simulink model "LIB_CoffeeMachine"  (R2024b)
settings: Solver=FixedStepAuto  StartTime=0.0  StopTime=10.0  FixedStep=0.1  RelTol=1e-3
libraries: simulink_extras x1
settings Model: Creator=RAPQ2Y  LastModifiedBy=RAPQ2Y
settings HardwareCC: ProdBitPerPointer=32  ProdBitPerSizeT=32  ProdBitPerPtrDiffT=32  ProdWordSize=32  ProdLongLongMode=on  ProdHWDeviceType=PHOENIX CONTACT->Generic PLCnext 32bit  TargetPreprocMaxBitsSint=64  TargetPreprocMaxBitsUint=64
settings SFSimCC: MATLABDynamicMemAlloc=off
settings RTWCC: Description=PLCnext Target for Simulink for GRT purpose  SystemTargetFile=pxc_plcn.tlc  TLCOptions=-m1 -p10000000000000000000  TemplateMakefile=pxc_plcn__2020b.tmf  TargetLang=C++
settings CodeAppCC: MaxIdLength=63
settings STFCustomTargetCC: TargetLibSuffix=.a  TargetLangStandard=C++03 (ISO)  CodeReplacementLibrary=GNU C99 extensions  ParMdlRefBuildCompliant=on  ConcurrentExecutionCompliant=on  CombineOutputUpdateFcns=on  SystemTargetFile=pxc_plcn.tlc
settings GRTTargetCC: TargetLibSuffix=.a  TargetLangStandard=C++03 (ISO)  CodeReplacementLibrary=GNU C99 extensions  CompOptLevelCompliant=off  MatFileLogging=off  CPPClassGenCompliant=off  UseToolchainInfoCompliant=off  ExtModeMexFile=ext_comm_plcn

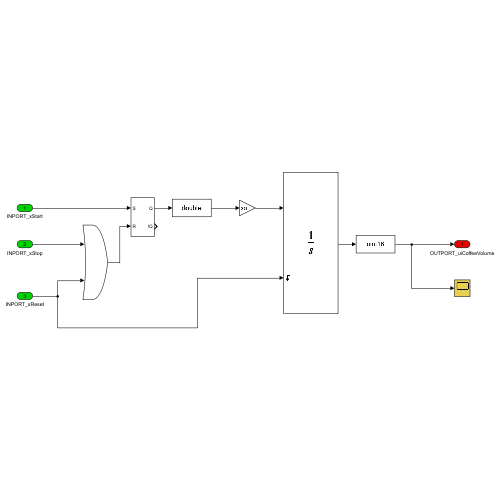
[thumbnail: Simulink's stored preview of the top-level diagram]
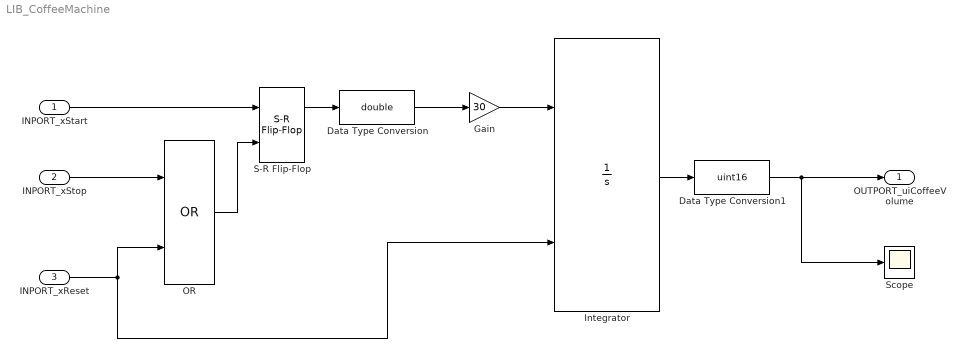
== system LIB_CoffeeMachine ==
  INPORT_xStart : Inport  OutDataTypeStr=boolean
  INPORT_xStop : Inport  Port=2  OutDataTypeStr=boolean
  INPORT_xReset : Inport  Port=3  OutDataTypeStr=boolean
  Data Type Conversion : DataTypeConversion  OutDataTypeStr=double  SaturateOnIntegerOverflow=off  RndMeth=Floor
  Data Type Conversion1 : DataTypeConversion  OutDataTypeStr=uint16  SaturateOnIntegerOverflow=off  RndMeth=Floor
  Gain : Gain  Gain=30
  Integrator : Integrator  ExternalReset=rising
  OR : Logic  Operator=OR  IconShape=distinctive  AllPortsSameDT=off  OutDataTypeStr=boolean
  S-R Flip-Flop : simulink_extras/Flip Flops/S-R Flip-Flop  initial_condition=0
  Scope : Scope
  OUTPORT_uiCoffeeVolume : Outport  OutDataTypeStr=uint16
  wires:
  Data Type Conversion1/1 -> Scope/1, OUTPORT_uiCoffeeVolume/1
  Data Type Conversion/1 -> Gain/1
  OR/1 -> S-R Flip-Flop/2
  INPORT_xStart/1 -> S-R Flip-Flop/1
  Integrator/1 -> Data Type Conversion1/1
  INPORT_xReset/1 -> Integrator/2, OR/2
  Gain/1 -> Integrator/1
  INPORT_xStop/1 -> OR/1
  S-R Flip-Flop/1 -> Data Type Conversion/1
